simulink model "TST_AirHt_Ctl"  (R2016b)
settings: Solver=FixedStepDiscrete  StartTime=0.0  StopTime=simTime  FixedStep=sampleTime  RelTol=1e-3
values from neighbouring files (symbols this model uses):
  testCase = 1    [initTST_AirHt_Ctl_001.m]    (also in initTST_AirHt_Ctl_002.m = 2; initTST_AirHt_Ctl_003.m = 3; initTST_AirHt_Ctl_004.m = 4; initTST_AirHt_Ctl_005.m = 5)
libraries: simulink x53, UnitTest_Lib x26
(part 2 of 4)

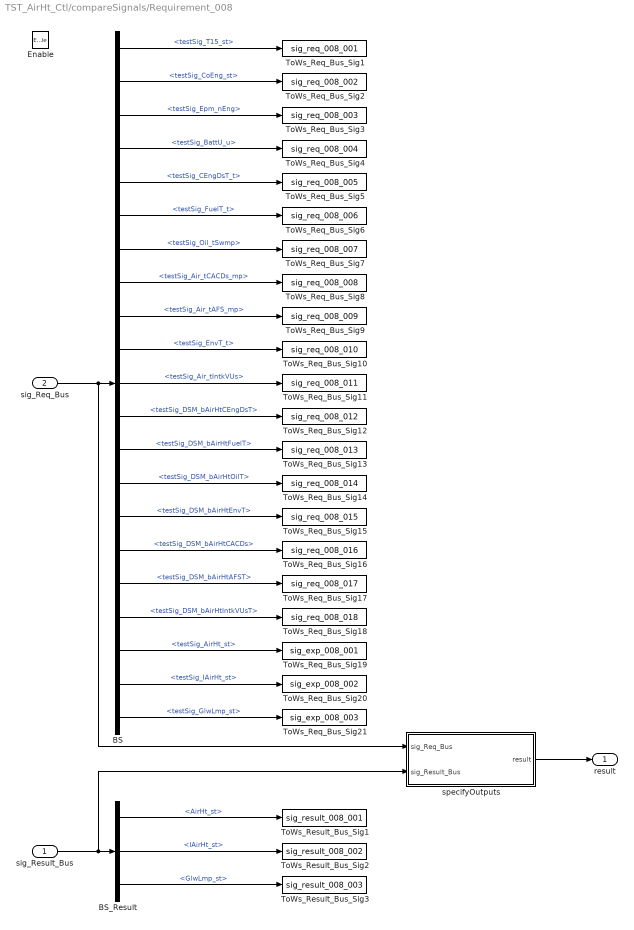
== system TST_AirHt_Ctl/compareSignals/Requirement_008 ==
  sig_Result_Bus : Inport
  sig_Req_Bus : Inport  Port=2
  Enable : EnablePort
  BS : BusSelector  OutputSignals=testSig_T15_st,testSig_CoEng_st,testSig_Epm_nEng,testSig_BattU_u,testSig_CEngDsT_t,testSig_FuelT_t,testSig_Oil_tSwmp,testSig_Air_tCACDs_mp,testSig_Air_tAFS_mp,testSig_EnvT_t,testSig_Air_tIntkVUs,testSig_DSM_bAirHtCEngDsT,testSig_DSM_bAirHtFuelT,testSig_DSM_bAirHtOilT,testSig_DSM_bAirHtEnvT,testSig_DSM_bAirHtCACDs,testSig_DSM_bAirHtAFST,testSig_DSM_bAirHtIntkVUsT,testSig_AirHt_st,testSig_IAirHt_st,testSig_GlwLmp_st
  BS_Result : BusSelector  OutputSignals=AirHt_st,IAirHt_st,GlwLmp_st
  ToWs_Req_Bus_Sig1 : ToWorkspace  VariableName=sig_req_008_001  SaveFormat=Structure With Time
  ToWs_Req_Bus_Sig10 : ToWorkspace  VariableName=sig_req_008_010  SaveFormat=Structure With Time
  ToWs_Req_Bus_Sig11 : ToWorkspace  VariableName=sig_req_008_011  SaveFormat=Structure With Time
  ToWs_Req_Bus_Sig12 : ToWorkspace  VariableName=sig_req_008_012  SaveFormat=Structure With Time
  ToWs_Req_Bus_Sig13 : ToWorkspace  VariableName=sig_req_008_013  SaveFormat=Structure With Time
  ToWs_Req_Bus_Sig14 : ToWorkspace  VariableName=sig_req_008_014  SaveFormat=Structure With Time
  ToWs_Req_Bus_Sig15 : ToWorkspace  VariableName=sig_req_008_015  SaveFormat=Structure With Time
  ToWs_Req_Bus_Sig16 : ToWorkspace  VariableName=sig_req_008_016  SaveFormat=Structure With Time
  ToWs_Req_Bus_Sig17 : ToWorkspace  VariableName=sig_req_008_017  SaveFormat=Structure With Time
  ToWs_Req_Bus_Sig18 : ToWorkspace  VariableName=sig_req_008_018  SaveFormat=Structure With Time
  ToWs_Req_Bus_Sig19 : ToWorkspace  VariableName=sig_exp_008_001  SaveFormat=Structure With Time
  ToWs_Req_Bus_Sig2 : ToWorkspace  VariableName=sig_req_008_002  SaveFormat=Structure With Time
  ToWs_Req_Bus_Sig20 : ToWorkspace  VariableName=sig_exp_008_002  SaveFormat=Structure With Time
  ToWs_Req_Bus_Sig21 : ToWorkspace  VariableName=sig_exp_008_003  SaveFormat=Structure With Time
  ToWs_Req_Bus_Sig3 : ToWorkspace  VariableName=sig_req_008_003  SaveFormat=Structure With Time
  ToWs_Req_Bus_Sig4 : ToWorkspace  VariableName=sig_req_008_004  SaveFormat=Structure With Time
  ToWs_Req_Bus_Sig5 : ToWorkspace  VariableName=sig_req_008_005  SaveFormat=Structure With Time
  ToWs_Req_Bus_Sig6 : ToWorkspace  VariableName=sig_req_008_006  SaveFormat=Structure With Time
  ToWs_Req_Bus_Sig7 : ToWorkspace  VariableName=sig_req_008_007  SaveFormat=Structure With Time
  ToWs_Req_Bus_Sig8 : ToWorkspace  VariableName=sig_req_008_008  SaveFormat=Structure With Time
  ToWs_Req_Bus_Sig9 : ToWorkspace  VariableName=sig_req_008_009  SaveFormat=Structure With Time
  ToWs_Result_Bus_Sig1 : ToWorkspace  VariableName=sig_result_008_001  SaveFormat=Structure With Time
  ToWs_Result_Bus_Sig2 : ToWorkspace  VariableName=sig_result_008_002  SaveFormat=Structure With Time
  ToWs_Result_Bus_Sig3 : ToWorkspace  VariableName=sig_result_008_003  SaveFormat=Structure With Time
  specifyOutputs : Subsystem
  result : Outport
  wires:
  sig_Req_Bus/1 -> BS/1, specifyOutputs/1(sig_Req_Bus)
  BS/1 -> ToWs_Req_Bus_Sig1/1  "<testSig_T15_st>"
  BS/2 -> ToWs_Req_Bus_Sig2/1  "<testSig_CoEng_st>"
  BS/3 -> ToWs_Req_Bus_Sig3/1  "<testSig_Epm_nEng>"
  BS/4 -> ToWs_Req_Bus_Sig4/1  "<testSig_BattU_u>"
  BS/5 -> ToWs_Req_Bus_Sig5/1  "<testSig_CEngDsT_t>"
  BS/6 -> ToWs_Req_Bus_Sig6/1  "<testSig_FuelT_t>"
  BS/7 -> ToWs_Req_Bus_Sig7/1  "<testSig_Oil_tSwmp>"
  BS/8 -> ToWs_Req_Bus_Sig8/1  "<testSig_Air_tCACDs_mp>"
  BS/9 -> ToWs_Req_Bus_Sig9/1  "<testSig_Air_tAFS_mp>"
  BS/10 -> ToWs_Req_Bus_Sig10/1  "<testSig_EnvT_t>"
  BS/11 -> ToWs_Req_Bus_Sig11/1  "<testSig_Air_tIntkVUs>"
  BS/12 -> ToWs_Req_Bus_Sig12/1  "<testSig_DSM_bAirHtCEngDsT>"
  BS/13 -> ToWs_Req_Bus_Sig13/1  "<testSig_DSM_bAirHtFuelT>"
  BS/14 -> ToWs_Req_Bus_Sig14/1  "<testSig_DSM_bAirHtOilT>"
  BS/15 -> ToWs_Req_Bus_Sig15/1  "<testSig_DSM_bAirHtEnvT>"
  BS/16 -> ToWs_Req_Bus_Sig16/1  "<testSig_DSM_bAirHtCACDs>"
  BS/17 -> ToWs_Req_Bus_Sig17/1  "<testSig_DSM_bAirHtAFST>"
  BS/18 -> ToWs_Req_Bus_Sig18/1  "<testSig_DSM_bAirHtIntkVUsT>"
  BS/19 -> ToWs_Req_Bus_Sig19/1  "<testSig_AirHt_st>"
  BS/20 -> ToWs_Req_Bus_Sig20/1  "<testSig_IAirHt_st>"
  BS/21 -> ToWs_Req_Bus_Sig21/1  "<testSig_GlwLmp_st>"
  sig_Result_Bus/1 -> BS_Result/1, specifyOutputs/2(sig_Result_Bus)
  BS_Result/1 -> ToWs_Result_Bus_Sig1/1  "<AirHt_st>"
  BS_Result/2 -> ToWs_Result_Bus_Sig2/1  "<IAirHt_st>"
  BS_Result/3 -> ToWs_Result_Bus_Sig3/1  "<GlwLmp_st>"
  specifyOutputs/1(result) -> result/1

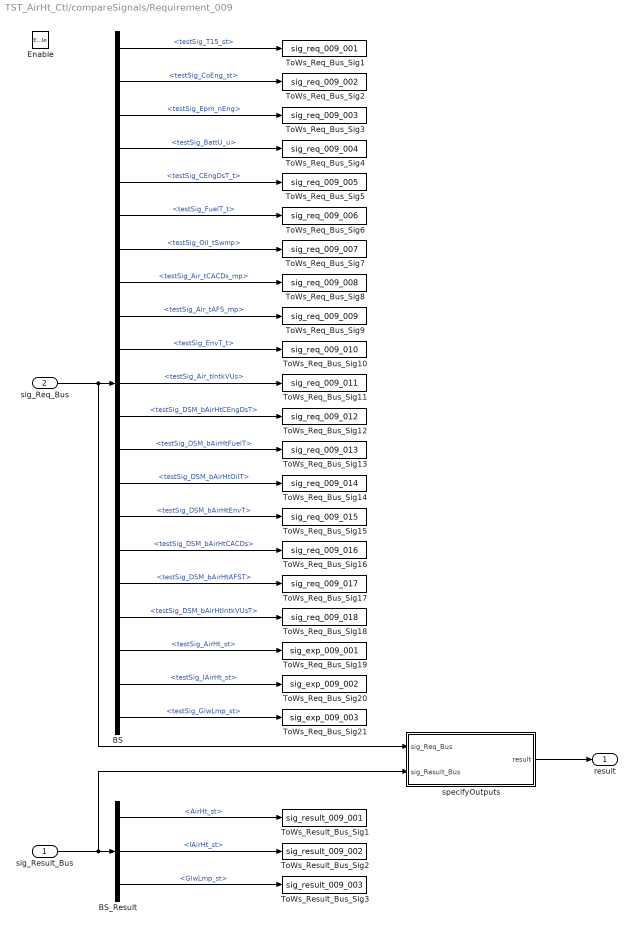
== system TST_AirHt_Ctl/compareSignals/Requirement_009 ==
  sig_Result_Bus : Inport
  sig_Req_Bus : Inport  Port=2
  Enable : EnablePort
  BS : BusSelector  OutputSignals=testSig_T15_st,testSig_CoEng_st,testSig_Epm_nEng,testSig_BattU_u,testSig_CEngDsT_t,testSig_FuelT_t,testSig_Oil_tSwmp,testSig_Air_tCACDs_mp,testSig_Air_tAFS_mp,testSig_EnvT_t,testSig_Air_tIntkVUs,testSig_DSM_bAirHtCEngDsT,testSig_DSM_bAirHtFuelT,testSig_DSM_bAirHtOilT,testSig_DSM_bAirHtEnvT,testSig_DSM_bAirHtCACDs,testSig_DSM_bAirHtAFST,testSig_DSM_bAirHtIntkVUsT,testSig_AirHt_st,testSig_IAirHt_st,testSig_GlwLmp_st
  BS_Result : BusSelector  OutputSignals=AirHt_st,IAirHt_st,GlwLmp_st
  ToWs_Req_Bus_Sig1 : ToWorkspace  VariableName=sig_req_009_001  SaveFormat=Structure With Time
  ToWs_Req_Bus_Sig10 : ToWorkspace  VariableName=sig_req_009_010  SaveFormat=Structure With Time
  ToWs_Req_Bus_Sig11 : ToWorkspace  VariableName=sig_req_009_011  SaveFormat=Structure With Time
  ToWs_Req_Bus_Sig12 : ToWorkspace  VariableName=sig_req_009_012  SaveFormat=Structure With Time
  ToWs_Req_Bus_Sig13 : ToWorkspace  VariableName=sig_req_009_013  SaveFormat=Structure With Time
  ToWs_Req_Bus_Sig14 : ToWorkspace  VariableName=sig_req_009_014  SaveFormat=Structure With Time
  ToWs_Req_Bus_Sig15 : ToWorkspace  VariableName=sig_req_009_015  SaveFormat=Structure With Time
  ToWs_Req_Bus_Sig16 : ToWorkspace  VariableName=sig_req_009_016  SaveFormat=Structure With Time
  ToWs_Req_Bus_Sig17 : ToWorkspace  VariableName=sig_req_009_017  SaveFormat=Structure With Time
  ToWs_Req_Bus_Sig18 : ToWorkspace  VariableName=sig_req_009_018  SaveFormat=Structure With Time
  ToWs_Req_Bus_Sig19 : ToWorkspace  VariableName=sig_exp_009_001  SaveFormat=Structure With Time
  ToWs_Req_Bus_Sig2 : ToWorkspace  VariableName=sig_req_009_002  SaveFormat=Structure With Time
  ToWs_Req_Bus_Sig20 : ToWorkspace  VariableName=sig_exp_009_002  SaveFormat=Structure With Time
  ToWs_Req_Bus_Sig21 : ToWorkspace  VariableName=sig_exp_009_003  SaveFormat=Structure With Time
  ToWs_Req_Bus_Sig3 : ToWorkspace  VariableName=sig_req_009_003  SaveFormat=Structure With Time
  ToWs_Req_Bus_Sig4 : ToWorkspace  VariableName=sig_req_009_004  SaveFormat=Structure With Time
  ToWs_Req_Bus_Sig5 : ToWorkspace  VariableName=sig_req_009_005  SaveFormat=Structure With Time
  ToWs_Req_Bus_Sig6 : ToWorkspace  VariableName=sig_req_009_006  SaveFormat=Structure With Time
  ToWs_Req_Bus_Sig7 : ToWorkspace  VariableName=sig_req_009_007  SaveFormat=Structure With Time
  ToWs_Req_Bus_Sig8 : ToWorkspace  VariableName=sig_req_009_008  SaveFormat=Structure With Time
  ToWs_Req_Bus_Sig9 : ToWorkspace  VariableName=sig_req_009_009  SaveFormat=Structure With Time
  ToWs_Result_Bus_Sig1 : ToWorkspace  VariableName=sig_result_009_001  SaveFormat=Structure With Time
  ToWs_Result_Bus_Sig2 : ToWorkspace  VariableName=sig_result_009_002  SaveFormat=Structure With Time
  ToWs_Result_Bus_Sig3 : ToWorkspace  VariableName=sig_result_009_003  SaveFormat=Structure With Time
  specifyOutputs : Subsystem
  result : Outport
  wires:
  sig_Req_Bus/1 -> BS/1, specifyOutputs/1(sig_Req_Bus)
  BS/1 -> ToWs_Req_Bus_Sig1/1  "<testSig_T15_st>"
  BS/2 -> ToWs_Req_Bus_Sig2/1  "<testSig_CoEng_st>"
  BS/3 -> ToWs_Req_Bus_Sig3/1  "<testSig_Epm_nEng>"
  BS/4 -> ToWs_Req_Bus_Sig4/1  "<testSig_BattU_u>"
  BS/5 -> ToWs_Req_Bus_Sig5/1  "<testSig_CEngDsT_t>"
  BS/6 -> ToWs_Req_Bus_Sig6/1  "<testSig_FuelT_t>"
  BS/7 -> ToWs_Req_Bus_Sig7/1  "<testSig_Oil_tSwmp>"
  BS/8 -> ToWs_Req_Bus_Sig8/1  "<testSig_Air_tCACDs_mp>"
  BS/9 -> ToWs_Req_Bus_Sig9/1  "<testSig_Air_tAFS_mp>"
  BS/10 -> ToWs_Req_Bus_Sig10/1  "<testSig_EnvT_t>"
  BS/11 -> ToWs_Req_Bus_Sig11/1  "<testSig_Air_tIntkVUs>"
  BS/12 -> ToWs_Req_Bus_Sig12/1  "<testSig_DSM_bAirHtCEngDsT>"
  BS/13 -> ToWs_Req_Bus_Sig13/1  "<testSig_DSM_bAirHtFuelT>"
  BS/14 -> ToWs_Req_Bus_Sig14/1  "<testSig_DSM_bAirHtOilT>"
  BS/15 -> ToWs_Req_Bus_Sig15/1  "<testSig_DSM_bAirHtEnvT>"
  BS/16 -> ToWs_Req_Bus_Sig16/1  "<testSig_DSM_bAirHtCACDs>"
  BS/17 -> ToWs_Req_Bus_Sig17/1  "<testSig_DSM_bAirHtAFST>"
  BS/18 -> ToWs_Req_Bus_Sig18/1  "<testSig_DSM_bAirHtIntkVUsT>"
  BS/19 -> ToWs_Req_Bus_Sig19/1  "<testSig_AirHt_st>"
  BS/20 -> ToWs_Req_Bus_Sig20/1  "<testSig_IAirHt_st>"
  BS/21 -> ToWs_Req_Bus_Sig21/1  "<testSig_GlwLmp_st>"
  sig_Result_Bus/1 -> BS_Result/1, specifyOutputs/2(sig_Result_Bus)
  BS_Result/1 -> ToWs_Result_Bus_Sig1/1  "<AirHt_st>"
  BS_Result/2 -> ToWs_Result_Bus_Sig2/1  "<IAirHt_st>"
  BS_Result/3 -> ToWs_Result_Bus_Sig3/1  "<GlwLmp_st>"
  specifyOutputs/1(result) -> result/1

== system TST_AirHt_Ctl/compareSignals/Requirement_010 ==
  sig_Result_Bus : Inport
  sig_Req_Bus : Inport  Port=2
  Enable : EnablePort
  BS : BusSelector  OutputSignals=testSig_T15_st,testSig_CoEng_st,testSig_Epm_nEng,testSig_BattU_u,testSig_CEngDsT_t,testSig_FuelT_t,testSig_Oil_tSwmp,testSig_Air_tCACDs_mp,testSig_Air_tAFS_mp,testSig_EnvT_t,testSig_Air_tIntkVUs,testSig_DSM_bAirHtCEngDsT,testSig_DSM_bAirHtFuelT,testSig_DSM_bAirHtOilT,testSig_DSM_bAirHtEnvT,testSig_DSM_bAirHtCACDs,testSig_DSM_bAirHtAFST,testSig_DSM_bAirHtIntkVUsT,testSig_AirHt_st,testSig_IAirHt_st,testSig_GlwLmp_st
  BS_Result : BusSelector  OutputSignals=AirHt_st,IAirHt_st,GlwLmp_st
  ToWs_Req_Bus_Sig1 : ToWorkspace  VariableName=sig_req_010_001  SaveFormat=Structure With Time
  ToWs_Req_Bus_Sig10 : ToWorkspace  VariableName=sig_req_010_010  SaveFormat=Structure With Time
  ToWs_Req_Bus_Sig11 : ToWorkspace  VariableName=sig_req_010_011  SaveFormat=Structure With Time
  ToWs_Req_Bus_Sig12 : ToWorkspace  VariableName=sig_req_010_012  SaveFormat=Structure With Time
  ToWs_Req_Bus_Sig13 : ToWorkspace  VariableName=sig_req_010_013  SaveFormat=Structure With Time
  ToWs_Req_Bus_Sig14 : ToWorkspace  VariableName=sig_req_010_014  SaveFormat=Structure With Time
  ToWs_Req_Bus_Sig15 : ToWorkspace  VariableName=sig_req_010_015  SaveFormat=Structure With Time
  ToWs_Req_Bus_Sig16 : ToWorkspace  VariableName=sig_req_010_016  SaveFormat=Structure With Time
  ToWs_Req_Bus_Sig17 : ToWorkspace  VariableName=sig_req_010_017  SaveFormat=Structure With Time
  ToWs_Req_Bus_Sig18 : ToWorkspace  VariableName=sig_req_010_018  SaveFormat=Structure With Time
  ToWs_Req_Bus_Sig19 : ToWorkspace  VariableName=sig_exp_010_001  SaveFormat=Structure With Time
  ToWs_Req_Bus_Sig2 : ToWorkspace  VariableName=sig_req_010_002  SaveFormat=Structure With Time
  ToWs_Req_Bus_Sig20 : ToWorkspace  VariableName=sig_exp_010_002  SaveFormat=Structure With Time
  ToWs_Req_Bus_Sig21 : ToWorkspace  VariableName=sig_exp_010_003  SaveFormat=Structure With Time
  ToWs_Req_Bus_Sig3 : ToWorkspace  VariableName=sig_req_010_003  SaveFormat=Structure With Time
  ToWs_Req_Bus_Sig4 : ToWorkspace  VariableName=sig_req_010_004  SaveFormat=Structure With Time
  ToWs_Req_Bus_Sig5 : ToWorkspace  VariableName=sig_req_010_005  SaveFormat=Structure With Time
  ToWs_Req_Bus_Sig6 : ToWorkspace  VariableName=sig_req_010_006  SaveFormat=Structure With Time
  ToWs_Req_Bus_Sig7 : ToWorkspace  VariableName=sig_req_010_007  SaveFormat=Structure With Time
  ToWs_Req_Bus_Sig8 : ToWorkspace  VariableName=sig_req_010_008  SaveFormat=Structure With Time
  ToWs_Req_Bus_Sig9 : ToWorkspace  VariableName=sig_req_010_009  SaveFormat=Structure With Time
  ToWs_Result_Bus_Sig1 : ToWorkspace  VariableName=sig_result_010_001  SaveFormat=Structure With Time
  ToWs_Result_Bus_Sig2 : ToWorkspace  VariableName=sig_result_010_002  SaveFormat=Structure With Time
  ToWs_Result_Bus_Sig3 : ToWorkspace  VariableName=sig_result_010_003  SaveFormat=Structure With Time
  specifyOutputs : Subsystem
  result : Outport
  wires:
  sig_Req_Bus/1 -> BS/1, specifyOutputs/1(sig_Req_Bus)
  BS/1 -> ToWs_Req_Bus_Sig1/1  "<testSig_T15_st>"
  BS/2 -> ToWs_Req_Bus_Sig2/1  "<testSig_CoEng_st>"
  BS/3 -> ToWs_Req_Bus_Sig3/1  "<testSig_Epm_nEng>"
  BS/4 -> ToWs_Req_Bus_Sig4/1  "<testSig_BattU_u>"
  BS/5 -> ToWs_Req_Bus_Sig5/1  "<testSig_CEngDsT_t>"
  BS/6 -> ToWs_Req_Bus_Sig6/1  "<testSig_FuelT_t>"
  BS/7 -> ToWs_Req_Bus_Sig7/1  "<testSig_Oil_tSwmp>"
  BS/8 -> ToWs_Req_Bus_Sig8/1  "<testSig_Air_tCACDs_mp>"
  BS/9 -> ToWs_Req_Bus_Sig9/1  "<testSig_Air_tAFS_mp>"
  BS/10 -> ToWs_Req_Bus_Sig10/1  "<testSig_EnvT_t>"
  BS/11 -> ToWs_Req_Bus_Sig11/1  "<testSig_Air_tIntkVUs>"
  BS/12 -> ToWs_Req_Bus_Sig12/1  "<testSig_DSM_bAirHtCEngDsT>"
  BS/13 -> ToWs_Req_Bus_Sig13/1  "<testSig_DSM_bAirHtFuelT>"
  BS/14 -> ToWs_Req_Bus_Sig14/1  "<testSig_DSM_bAirHtOilT>"
  BS/15 -> ToWs_Req_Bus_Sig15/1  "<testSig_DSM_bAirHtEnvT>"
  BS/16 -> ToWs_Req_Bus_Sig16/1  "<testSig_DSM_bAirHtCACDs>"
  BS/17 -> ToWs_Req_Bus_Sig17/1  "<testSig_DSM_bAirHtAFST>"
  BS/18 -> ToWs_Req_Bus_Sig18/1  "<testSig_DSM_bAirHtIntkVUsT>"
  BS/19 -> ToWs_Req_Bus_Sig19/1  "<testSig_AirHt_st>"
  BS/20 -> ToWs_Req_Bus_Sig20/1  "<testSig_IAirHt_st>"
  BS/21 -> ToWs_Req_Bus_Sig21/1  "<testSig_GlwLmp_st>"
  sig_Result_Bus/1 -> BS_Result/1, specifyOutputs/2(sig_Result_Bus)
  BS_Result/1 -> ToWs_Result_Bus_Sig1/1  "<AirHt_st>"
  BS_Result/2 -> ToWs_Result_Bus_Sig2/1  "<IAirHt_st>"
  BS_Result/3 -> ToWs_Result_Bus_Sig3/1  "<GlwLmp_st>"
  specifyOutputs/1(result) -> result/1

== system TST_AirHt_Ctl/compareSignals/Requirement_011 ==
  sig_Result_Bus : Inport
  sig_Req_Bus : Inport  Port=2
  Enable : EnablePort
  BS : BusSelector  OutputSignals=testSig_T15_st,testSig_CoEng_st,testSig_Epm_nEng,testSig_BattU_u,testSig_CEngDsT_t,testSig_FuelT_t,testSig_Oil_tSwmp,testSig_Air_tCACDs_mp,testSig_Air_tAFS_mp,testSig_EnvT_t,testSig_Air_tIntkVUs,testSig_DSM_bAirHtCEngDsT,testSig_DSM_bAirHtFuelT,testSig_DSM_bAirHtOilT,testSig_DSM_bAirHtEnvT,testSig_DSM_bAirHtCACDs,testSig_DSM_bAirHtAFST,testSig_DSM_bAirHtIntkVUsT,testSig_AirHt_st,testSig_IAirHt_st,testSig_GlwLmp_st
  BS_Result : BusSelector  OutputSignals=AirHt_st,IAirHt_st,GlwLmp_st
  ToWs_Req_Bus_Sig1 : ToWorkspace  VariableName=sig_req_011_001  SaveFormat=Structure With Time
  ToWs_Req_Bus_Sig10 : ToWorkspace  VariableName=sig_req_011_010  SaveFormat=Structure With Time
  ToWs_Req_Bus_Sig11 : ToWorkspace  VariableName=sig_req_011_011  SaveFormat=Structure With Time
  ToWs_Req_Bus_Sig12 : ToWorkspace  VariableName=sig_req_011_012  SaveFormat=Structure With Time
  ToWs_Req_Bus_Sig13 : ToWorkspace  VariableName=sig_req_011_013  SaveFormat=Structure With Time
  ToWs_Req_Bus_Sig14 : ToWorkspace  VariableName=sig_req_011_014  SaveFormat=Structure With Time
  ToWs_Req_Bus_Sig15 : ToWorkspace  VariableName=sig_req_011_015  SaveFormat=Structure With Time
  ToWs_Req_Bus_Sig16 : ToWorkspace  VariableName=sig_req_011_016  SaveFormat=Structure With Time
  ToWs_Req_Bus_Sig17 : ToWorkspace  VariableName=sig_req_011_017  SaveFormat=Structure With Time
  ToWs_Req_Bus_Sig18 : ToWorkspace  VariableName=sig_req_011_018  SaveFormat=Structure With Time
  ToWs_Req_Bus_Sig19 : ToWorkspace  VariableName=sig_exp_011_001  SaveFormat=Structure With Time
  ToWs_Req_Bus_Sig2 : ToWorkspace  VariableName=sig_req_011_002  SaveFormat=Structure With Time
  ToWs_Req_Bus_Sig20 : ToWorkspace  VariableName=sig_exp_011_002  SaveFormat=Structure With Time
  ToWs_Req_Bus_Sig21 : ToWorkspace  VariableName=sig_exp_011_003  SaveFormat=Structure With Time
  ToWs_Req_Bus_Sig3 : ToWorkspace  VariableName=sig_req_011_003  SaveFormat=Structure With Time
  ToWs_Req_Bus_Sig4 : ToWorkspace  VariableName=sig_req_011_004  SaveFormat=Structure With Time
  ToWs_Req_Bus_Sig5 : ToWorkspace  VariableName=sig_req_011_005  SaveFormat=Structure With Time
  ToWs_Req_Bus_Sig6 : ToWorkspace  VariableName=sig_req_011_006  SaveFormat=Structure With Time
  ToWs_Req_Bus_Sig7 : ToWorkspace  VariableName=sig_req_011_007  SaveFormat=Structure With Time
  ToWs_Req_Bus_Sig8 : ToWorkspace  VariableName=sig_req_011_008  SaveFormat=Structure With Time
  ToWs_Req_Bus_Sig9 : ToWorkspace  VariableName=sig_req_011_009  SaveFormat=Structure With Time
  ToWs_Result_Bus_Sig1 : ToWorkspace  VariableName=sig_result_011_001  SaveFormat=Structure With Time
  ToWs_Result_Bus_Sig2 : ToWorkspace  VariableName=sig_result_011_002  SaveFormat=Structure With Time
  ToWs_Result_Bus_Sig3 : ToWorkspace  VariableName=sig_result_011_003  SaveFormat=Structure With Time
  specifyOutputs : Subsystem
  result : Outport
  wires:
  sig_Req_Bus/1 -> BS/1, specifyOutputs/1(sig_Req_Bus)
  BS/1 -> ToWs_Req_Bus_Sig1/1  "<testSig_T15_st>"
  BS/2 -> ToWs_Req_Bus_Sig2/1  "<testSig_CoEng_st>"
  BS/3 -> ToWs_Req_Bus_Sig3/1  "<testSig_Epm_nEng>"
  BS/4 -> ToWs_Req_Bus_Sig4/1  "<testSig_BattU_u>"
  BS/5 -> ToWs_Req_Bus_Sig5/1  "<testSig_CEngDsT_t>"
  BS/6 -> ToWs_Req_Bus_Sig6/1  "<testSig_FuelT_t>"
  BS/7 -> ToWs_Req_Bus_Sig7/1  "<testSig_Oil_tSwmp>"
  BS/8 -> ToWs_Req_Bus_Sig8/1  "<testSig_Air_tCACDs_mp>"
  BS/9 -> ToWs_Req_Bus_Sig9/1  "<testSig_Air_tAFS_mp>"
  BS/10 -> ToWs_Req_Bus_Sig10/1  "<testSig_EnvT_t>"
  BS/11 -> ToWs_Req_Bus_Sig11/1  "<testSig_Air_tIntkVUs>"
  BS/12 -> ToWs_Req_Bus_Sig12/1  "<testSig_DSM_bAirHtCEngDsT>"
  BS/13 -> ToWs_Req_Bus_Sig13/1  "<testSig_DSM_bAirHtFuelT>"
  BS/14 -> ToWs_Req_Bus_Sig14/1  "<testSig_DSM_bAirHtOilT>"
  BS/15 -> ToWs_Req_Bus_Sig15/1  "<testSig_DSM_bAirHtEnvT>"
  BS/16 -> ToWs_Req_Bus_Sig16/1  "<testSig_DSM_bAirHtCACDs>"
  BS/17 -> ToWs_Req_Bus_Sig17/1  "<testSig_DSM_bAirHtAFST>"
  BS/18 -> ToWs_Req_Bus_Sig18/1  "<testSig_DSM_bAirHtIntkVUsT>"
  BS/19 -> ToWs_Req_Bus_Sig19/1  "<testSig_AirHt_st>"
  BS/20 -> ToWs_Req_Bus_Sig20/1  "<testSig_IAirHt_st>"
  BS/21 -> ToWs_Req_Bus_Sig21/1  "<testSig_GlwLmp_st>"
  sig_Result_Bus/1 -> BS_Result/1, specifyOutputs/2(sig_Result_Bus)
  BS_Result/1 -> ToWs_Result_Bus_Sig1/1  "<AirHt_st>"
  BS_Result/2 -> ToWs_Result_Bus_Sig2/1  "<IAirHt_st>"
  BS_Result/3 -> ToWs_Result_Bus_Sig3/1  "<GlwLmp_st>"
  specifyOutputs/1(result) -> result/1

== system TST_AirHt_Ctl/compareSignals/Requirement_012 ==
  sig_Result_Bus : Inport
  sig_Req_Bus : Inport  Port=2
  Enable : EnablePort
  BS : BusSelector  OutputSignals=testSig_T15_st,testSig_CoEng_st,testSig_Epm_nEng,testSig_BattU_u,testSig_CEngDsT_t,testSig_FuelT_t,testSig_Oil_tSwmp,testSig_Air_tCACDs_mp,testSig_Air_tAFS_mp,testSig_EnvT_t,testSig_Air_tIntkVUs,testSig_DSM_bAirHtCEngDsT,testSig_DSM_bAirHtFuelT,testSig_DSM_bAirHtOilT,testSig_DSM_bAirHtEnvT,testSig_DSM_bAirHtCACDs,testSig_DSM_bAirHtAFST,testSig_DSM_bAirHtIntkVUsT,testSig_AirHt_st,testSig_IAirHt_st,testSig_GlwLmp_st
  BS_Result : BusSelector  OutputSignals=AirHt_st,IAirHt_st,GlwLmp_st
  ToWs_Req_Bus_Sig1 : ToWorkspace  VariableName=sig_req_012_001  SaveFormat=Structure With Time
  ToWs_Req_Bus_Sig10 : ToWorkspace  VariableName=sig_req_012_010  SaveFormat=Structure With Time
  ToWs_Req_Bus_Sig11 : ToWorkspace  VariableName=sig_req_012_011  SaveFormat=Structure With Time
  ToWs_Req_Bus_Sig12 : ToWorkspace  VariableName=sig_req_012_012  SaveFormat=Structure With Time
  ToWs_Req_Bus_Sig13 : ToWorkspace  VariableName=sig_req_012_013  SaveFormat=Structure With Time
  ToWs_Req_Bus_Sig14 : ToWorkspace  VariableName=sig_req_012_014  SaveFormat=Structure With Time
  ToWs_Req_Bus_Sig15 : ToWorkspace  VariableName=sig_req_012_015  SaveFormat=Structure With Time
  ToWs_Req_Bus_Sig16 : ToWorkspace  VariableName=sig_req_012_016  SaveFormat=Structure With Time
  ToWs_Req_Bus_Sig17 : ToWorkspace  VariableName=sig_req_012_017  SaveFormat=Structure With Time
  ToWs_Req_Bus_Sig18 : ToWorkspace  VariableName=sig_req_012_018  SaveFormat=Structure With Time
  ToWs_Req_Bus_Sig19 : ToWorkspace  VariableName=sig_exp_012_001  SaveFormat=Structure With Time
  ToWs_Req_Bus_Sig2 : ToWorkspace  VariableName=sig_req_012_002  SaveFormat=Structure With Time
  ToWs_Req_Bus_Sig20 : ToWorkspace  VariableName=sig_exp_012_002  SaveFormat=Structure With Time
  ToWs_Req_Bus_Sig21 : ToWorkspace  VariableName=sig_exp_012_003  SaveFormat=Structure With Time
  ToWs_Req_Bus_Sig3 : ToWorkspace  VariableName=sig_req_012_003  SaveFormat=Structure With Time
  ToWs_Req_Bus_Sig4 : ToWorkspace  VariableName=sig_req_012_004  SaveFormat=Structure With Time
  ToWs_Req_Bus_Sig5 : ToWorkspace  VariableName=sig_req_012_005  SaveFormat=Structure With Time
  ToWs_Req_Bus_Sig6 : ToWorkspace  VariableName=sig_req_012_006  SaveFormat=Structure With Time
  ToWs_Req_Bus_Sig7 : ToWorkspace  VariableName=sig_req_012_007  SaveFormat=Structure With Time
  ToWs_Req_Bus_Sig8 : ToWorkspace  VariableName=sig_req_012_008  SaveFormat=Structure With Time
  ToWs_Req_Bus_Sig9 : ToWorkspace  VariableName=sig_req_012_009  SaveFormat=Structure With Time
  ToWs_Result_Bus_Sig1 : ToWorkspace  VariableName=sig_result_012_001  SaveFormat=Structure With Time
  ToWs_Result_Bus_Sig2 : ToWorkspace  VariableName=sig_result_012_002  SaveFormat=Structure With Time
  ToWs_Result_Bus_Sig3 : ToWorkspace  VariableName=sig_result_012_003  SaveFormat=Structure With Time
  specifyOutputs : Subsystem
  result : Outport
  wires:
  sig_Req_Bus/1 -> BS/1, specifyOutputs/1(sig_Req_Bus)
  BS/1 -> ToWs_Req_Bus_Sig1/1  "<testSig_T15_st>"
  BS/2 -> ToWs_Req_Bus_Sig2/1  "<testSig_CoEng_st>"
  BS/3 -> ToWs_Req_Bus_Sig3/1  "<testSig_Epm_nEng>"
  BS/4 -> ToWs_Req_Bus_Sig4/1  "<testSig_BattU_u>"
  BS/5 -> ToWs_Req_Bus_Sig5/1  "<testSig_CEngDsT_t>"
  BS/6 -> ToWs_Req_Bus_Sig6/1  "<testSig_FuelT_t>"
  BS/7 -> ToWs_Req_Bus_Sig7/1  "<testSig_Oil_tSwmp>"
  BS/8 -> ToWs_Req_Bus_Sig8/1  "<testSig_Air_tCACDs_mp>"
  BS/9 -> ToWs_Req_Bus_Sig9/1  "<testSig_Air_tAFS_mp>"
  BS/10 -> ToWs_Req_Bus_Sig10/1  "<testSig_EnvT_t>"
  BS/11 -> ToWs_Req_Bus_Sig11/1  "<testSig_Air_tIntkVUs>"
  BS/12 -> ToWs_Req_Bus_Sig12/1  "<testSig_DSM_bAirHtCEngDsT>"
  BS/13 -> ToWs_Req_Bus_Sig13/1  "<testSig_DSM_bAirHtFuelT>"
  BS/14 -> ToWs_Req_Bus_Sig14/1  "<testSig_DSM_bAirHtOilT>"
  BS/15 -> ToWs_Req_Bus_Sig15/1  "<testSig_DSM_bAirHtEnvT>"
  BS/16 -> ToWs_Req_Bus_Sig16/1  "<testSig_DSM_bAirHtCACDs>"
  BS/17 -> ToWs_Req_Bus_Sig17/1  "<testSig_DSM_bAirHtAFST>"
  BS/18 -> ToWs_Req_Bus_Sig18/1  "<testSig_DSM_bAirHtIntkVUsT>"
  BS/19 -> ToWs_Req_Bus_Sig19/1  "<testSig_AirHt_st>"
  BS/20 -> ToWs_Req_Bus_Sig20/1  "<testSig_IAirHt_st>"
  BS/21 -> ToWs_Req_Bus_Sig21/1  "<testSig_GlwLmp_st>"
  sig_Result_Bus/1 -> BS_Result/1, specifyOutputs/2(sig_Result_Bus)
  BS_Result/1 -> ToWs_Result_Bus_Sig1/1  "<AirHt_st>"
  BS_Result/2 -> ToWs_Result_Bus_Sig2/1  "<IAirHt_st>"
  BS_Result/3 -> ToWs_Result_Bus_Sig3/1  "<GlwLmp_st>"
  specifyOutputs/1(result) -> result/1

== system TST_AirHt_Ctl/compareSignals/Requirement_013 ==
  sig_Result_Bus : Inport
  sig_Req_Bus : Inport  Port=2
  Enable : EnablePort
  BS : BusSelector  OutputSignals=testSig_T15_st,testSig_CoEng_st,testSig_Epm_nEng,testSig_BattU_u,testSig_CEngDsT_t,testSig_FuelT_t,testSig_Oil_tSwmp,testSig_Air_tCACDs_mp,testSig_Air_tAFS_mp,testSig_EnvT_t,testSig_Air_tIntkVUs,testSig_DSM_bAirHtCEngDsT,testSig_DSM_bAirHtFuelT,testSig_DSM_bAirHtOilT,testSig_DSM_bAirHtEnvT,testSig_DSM_bAirHtCACDs,testSig_DSM_bAirHtAFST,testSig_DSM_bAirHtIntkVUsT,testSig_AirHt_st,testSig_IAirHt_st,testSig_GlwLmp_st
  BS_Result : BusSelector  OutputSignals=AirHt_st,IAirHt_st,GlwLmp_st
  ToWs_Req_Bus_Sig1 : ToWorkspace  VariableName=sig_req_013_001  SaveFormat=Structure With Time
  ToWs_Req_Bus_Sig10 : ToWorkspace  VariableName=sig_req_013_010  SaveFormat=Structure With Time
  ToWs_Req_Bus_Sig11 : ToWorkspace  VariableName=sig_req_013_011  SaveFormat=Structure With Time
  ToWs_Req_Bus_Sig12 : ToWorkspace  VariableName=sig_req_013_012  SaveFormat=Structure With Time
  ToWs_Req_Bus_Sig13 : ToWorkspace  VariableName=sig_req_013_013  SaveFormat=Structure With Time
  ToWs_Req_Bus_Sig14 : ToWorkspace  VariableName=sig_req_013_014  SaveFormat=Structure With Time
  ToWs_Req_Bus_Sig15 : ToWorkspace  VariableName=sig_req_013_015  SaveFormat=Structure With Time
  ToWs_Req_Bus_Sig16 : ToWorkspace  VariableName=sig_req_013_016  SaveFormat=Structure With Time
  ToWs_Req_Bus_Sig17 : ToWorkspace  VariableName=sig_req_013_017  SaveFormat=Structure With Time
  ToWs_Req_Bus_Sig18 : ToWorkspace  VariableName=sig_req_013_018  SaveFormat=Structure With Time
  ToWs_Req_Bus_Sig19 : ToWorkspace  VariableName=sig_exp_013_001  SaveFormat=Structure With Time
  ToWs_Req_Bus_Sig2 : ToWorkspace  VariableName=sig_req_013_002  SaveFormat=Structure With Time
  ToWs_Req_Bus_Sig20 : ToWorkspace  VariableName=sig_exp_013_002  SaveFormat=Structure With Time
  ToWs_Req_Bus_Sig21 : ToWorkspace  VariableName=sig_exp_013_003  SaveFormat=Structure With Time
  ToWs_Req_Bus_Sig3 : ToWorkspace  VariableName=sig_req_013_003  SaveFormat=Structure With Time
  ToWs_Req_Bus_Sig4 : ToWorkspace  VariableName=sig_req_013_004  SaveFormat=Structure With Time
  ToWs_Req_Bus_Sig5 : ToWorkspace  VariableName=sig_req_013_005  SaveFormat=Structure With Time
  ToWs_Req_Bus_Sig6 : ToWorkspace  VariableName=sig_req_013_006  SaveFormat=Structure With Time
  ToWs_Req_Bus_Sig7 : ToWorkspace  VariableName=sig_req_013_007  SaveFormat=Structure With Time
  ToWs_Req_Bus_Sig8 : ToWorkspace  VariableName=sig_req_013_008  SaveFormat=Structure With Time
  ToWs_Req_Bus_Sig9 : ToWorkspace  VariableName=sig_req_013_009  SaveFormat=Structure With Time
  ToWs_Result_Bus_Sig1 : ToWorkspace  VariableName=sig_result_013_001  SaveFormat=Structure With Time
  ToWs_Result_Bus_Sig2 : ToWorkspace  VariableName=sig_result_013_002  SaveFormat=Structure With Time
  ToWs_Result_Bus_Sig3 : ToWorkspace  VariableName=sig_result_013_003  SaveFormat=Structure With Time
  specifyOutputs : Subsystem
  result : Outport
  wires:
  sig_Req_Bus/1 -> BS/1, specifyOutputs/1(sig_Req_Bus)
  BS/1 -> ToWs_Req_Bus_Sig1/1  "<testSig_T15_st>"
  BS/2 -> ToWs_Req_Bus_Sig2/1  "<testSig_CoEng_st>"
  BS/3 -> ToWs_Req_Bus_Sig3/1  "<testSig_Epm_nEng>"
  BS/4 -> ToWs_Req_Bus_Sig4/1  "<testSig_BattU_u>"
  BS/5 -> ToWs_Req_Bus_Sig5/1  "<testSig_CEngDsT_t>"
  BS/6 -> ToWs_Req_Bus_Sig6/1  "<testSig_FuelT_t>"
  BS/7 -> ToWs_Req_Bus_Sig7/1  "<testSig_Oil_tSwmp>"
  BS/8 -> ToWs_Req_Bus_Sig8/1  "<testSig_Air_tCACDs_mp>"
  BS/9 -> ToWs_Req_Bus_Sig9/1  "<testSig_Air_tAFS_mp>"
  BS/10 -> ToWs_Req_Bus_Sig10/1  "<testSig_EnvT_t>"
  BS/11 -> ToWs_Req_Bus_Sig11/1  "<testSig_Air_tIntkVUs>"
  BS/12 -> ToWs_Req_Bus_Sig12/1  "<testSig_DSM_bAirHtCEngDsT>"
  BS/13 -> ToWs_Req_Bus_Sig13/1  "<testSig_DSM_bAirHtFuelT>"
  BS/14 -> ToWs_Req_Bus_Sig14/1  "<testSig_DSM_bAirHtOilT>"
  BS/15 -> ToWs_Req_Bus_Sig15/1  "<testSig_DSM_bAirHtEnvT>"
  BS/16 -> ToWs_Req_Bus_Sig16/1  "<testSig_DSM_bAirHtCACDs>"
  BS/17 -> ToWs_Req_Bus_Sig17/1  "<testSig_DSM_bAirHtAFST>"
  BS/18 -> ToWs_Req_Bus_Sig18/1  "<testSig_DSM_bAirHtIntkVUsT>"
  BS/19 -> ToWs_Req_Bus_Sig19/1  "<testSig_AirHt_st>"
  BS/20 -> ToWs_Req_Bus_Sig20/1  "<testSig_IAirHt_st>"
  BS/21 -> ToWs_Req_Bus_Sig21/1  "<testSig_GlwLmp_st>"
  sig_Result_Bus/1 -> BS_Result/1, specifyOutputs/2(sig_Result_Bus)
  BS_Result/1 -> ToWs_Result_Bus_Sig1/1  "<AirHt_st>"
  BS_Result/2 -> ToWs_Result_Bus_Sig2/1  "<IAirHt_st>"
  BS_Result/3 -> ToWs_Result_Bus_Sig3/1  "<GlwLmp_st>"
  specifyOutputs/1(result) -> result/1

== system TST_AirHt_Ctl/simulationInput/testSignals_R001 ==
  BC : BusCreator  Inputs=21
  spec_AirHt_st : FromWorkspace  VariableName=testSig_AirHt_st  Interpolate=off  OutputAfterFinalValue=Holding final value
  spec_Air_tAFS_mp : FromWorkspace  VariableName=testSig_Air_tAFS_mp  Interpolate=off  OutputAfterFinalValue=Holding final value
  spec_Air_tCACDs_mp : FromWorkspace  VariableName=testSig_Air_tCACDs_mp  Interpolate=off  OutputAfterFinalValue=Holding final value
  spec_Air_tIntkVUs : FromWorkspace  VariableName=testSig_Air_tIntkVUs  Interpolate=off  OutputAfterFinalValue=Holding final value
  spec_BattU_u : FromWorkspace  VariableName=testSig_BattU_u  Interpolate=off  OutputAfterFinalValue=Holding final value
  spec_CEngDsT_t : FromWorkspace  VariableName=testSig_CEngDsT_t  Interpolate=off  OutputAfterFinalValue=Holding final value
  spec_CoEng_st : FromWorkspace  VariableName=testSig_CoEng_st  Interpolate=off  OutputAfterFinalValue=Holding final value
  spec_DSM_bAirHtAFST : FromWorkspace  VariableName=testSig_DSM_bAirHtAFST  Interpolate=off  OutputAfterFinalValue=Holding final value
  spec_DSM_bAirHtCACDs : FromWorkspace  VariableName=testSig_DSM_bAirHtCACDs  Interpolate=off  OutputAfterFinalValue=Holding final value
  spec_DSM_bAirHtCEngDsT : FromWorkspace  VariableName=testSig_DSM_bAirHtCEngDsT  Interpolate=off  OutputAfterFinalValue=Holding final value
  spec_DSM_bAirHtEnvT : FromWorkspace  VariableName=testSig_DSM_bAirHtEnvT  Interpolate=off  OutputAfterFinalValue=Holding final value
  spec_DSM_bAirHtFuelT : FromWorkspace  VariableName=testSig_DSM_bAirHtFuelT  Interpolate=off  OutputAfterFinalValue=Holding final value
  spec_DSM_bAirHtIntkVUsT : FromWorkspace  VariableName=testSig_DSM_bAirHtIntkVUsT  Interpolate=off  OutputAfterFinalValue=Holding final value
  spec_DSM_bAirHtOilT : FromWorkspace  VariableName=testSig_DSM_bAirHtOilT  Interpolate=off  OutputAfterFinalValue=Holding final value
  spec_EnvT_t : FromWorkspace  VariableName=testSig_EnvT_t  Interpolate=off  OutputAfterFinalValue=Holding final value
  spec_Epm_nEng : FromWorkspace  VariableName=testSig_Epm_nEng  Interpolate=off  OutputAfterFinalValue=Holding final value
  spec_FuelT_t : FromWorkspace  VariableName=testSig_FuelT_t  Interpolate=off  OutputAfterFinalValue=Holding final value
  spec_GlwLmp_st : FromWorkspace  VariableName=testSig_GlwLmp_st  Interpolate=off  OutputAfterFinalValue=Holding final value
  spec_IAirHt_st : FromWorkspace  VariableName=testSig_IAirHt_st  Interpolate=off  OutputAfterFinalValue=Holding final value
  spec_Oil_tSwmp : FromWorkspace  VariableName=testSig_Oil_tSwmp  Interpolate=off  OutputAfterFinalValue=Holding final value
  spec_T15_st : FromWorkspace  VariableName=testSig_T15_st  Interpolate=off  OutputAfterFinalValue=Holding final value
  testSignals : Outport
  wires:
  BC/1 -> testSignals/1
  spec_T15_st/1 -> BC/1  "testSig_T15_st"
  spec_CoEng_st/1 -> BC/2  "testSig_CoEng_st"
  spec_Epm_nEng/1 -> BC/3  "testSig_Epm_nEng"
  spec_BattU_u/1 -> BC/4  "testSig_BattU_u"
  spec_CEngDsT_t/1 -> BC/5  "testSig_CEngDsT_t"
  spec_FuelT_t/1 -> BC/6  "testSig_FuelT_t"
  spec_Oil_tSwmp/1 -> BC/7  "testSig_Oil_tSwmp"
  spec_Air_tCACDs_mp/1 -> BC/8  "testSig_Air_tCACDs_mp"
  spec_Air_tAFS_mp/1 -> BC/9  "testSig_Air_tAFS_mp"
  spec_EnvT_t/1 -> BC/10  "testSig_EnvT_t"
  spec_Air_tIntkVUs/1 -> BC/11  "testSig_Air_tIntkVUs"
  spec_DSM_bAirHtCEngDsT/1 -> BC/12  "testSig_DSM_bAirHtCEngDsT"
  spec_DSM_bAirHtFuelT/1 -> BC/13  "testSig_DSM_bAirHtFuelT"
  spec_DSM_bAirHtOilT/1 -> BC/14  "testSig_DSM_bAirHtOilT"
  spec_DSM_bAirHtEnvT/1 -> BC/15  "testSig_DSM_bAirHtEnvT"
  spec_DSM_bAirHtCACDs/1 -> BC/16  "testSig_DSM_bAirHtCACDs"
  spec_DSM_bAirHtAFST/1 -> BC/17  "testSig_DSM_bAirHtAFST"
  spec_DSM_bAirHtIntkVUsT/1 -> BC/18  "testSig_DSM_bAirHtIntkVUsT"
  spec_AirHt_st/1 -> BC/19  "testSig_AirHt_st"
  spec_IAirHt_st/1 -> BC/20  "testSig_IAirHt_st"
  spec_GlwLmp_st/1 -> BC/21  "testSig_GlwLmp_st"

== system TST_AirHt_Ctl/simulationInput/testSignals_R002 ==
  BC : BusCreator  Inputs=21
  spec_AirHt_st : FromWorkspace  VariableName=testSig_AirHt_st  Interpolate=off  OutputAfterFinalValue=Holding final value
  spec_Air_tAFS_mp : FromWorkspace  VariableName=testSig_Air_tAFS_mp  Interpolate=off  OutputAfterFinalValue=Holding final value
  spec_Air_tCACDs_mp : FromWorkspace  VariableName=testSig_Air_tCACDs_mp  Interpolate=off  OutputAfterFinalValue=Holding final value
  spec_Air_tIntkVUs : FromWorkspace  VariableName=testSig_Air_tIntkVUs  Interpolate=off  OutputAfterFinalValue=Holding final value
  spec_BattU_u : FromWorkspace  VariableName=testSig_BattU_u  Interpolate=off  OutputAfterFinalValue=Holding final value
  spec_CEngDsT_t : FromWorkspace  VariableName=testSig_CEngDsT_t  Interpolate=off  OutputAfterFinalValue=Holding final value
  spec_CoEng_st : FromWorkspace  VariableName=testSig_CoEng_st  Interpolate=off  OutputAfterFinalValue=Holding final value
  spec_DSM_bAirHtAFST : FromWorkspace  VariableName=testSig_DSM_bAirHtAFST  Interpolate=off  OutputAfterFinalValue=Holding final value
  spec_DSM_bAirHtCACDs : FromWorkspace  VariableName=testSig_DSM_bAirHtCACDs  Interpolate=off  OutputAfterFinalValue=Holding final value
  spec_DSM_bAirHtCEngDsT : FromWorkspace  VariableName=testSig_DSM_bAirHtCEngDsT  Interpolate=off  OutputAfterFinalValue=Holding final value
  spec_DSM_bAirHtEnvT : FromWorkspace  VariableName=testSig_DSM_bAirHtEnvT  Interpolate=off  OutputAfterFinalValue=Holding final value
  spec_DSM_bAirHtFuelT : FromWorkspace  VariableName=testSig_DSM_bAirHtFuelT  Interpolate=off  OutputAfterFinalValue=Holding final value
  spec_DSM_bAirHtIntkVUsT : FromWorkspace  VariableName=testSig_DSM_bAirHtIntkVUsT  Interpolate=off  OutputAfterFinalValue=Holding final value
  spec_DSM_bAirHtOilT : FromWorkspace  VariableName=testSig_DSM_bAirHtOilT  Interpolate=off  OutputAfterFinalValue=Holding final value
  spec_EnvT_t : FromWorkspace  VariableName=testSig_EnvT_t  Interpolate=off  OutputAfterFinalValue=Holding final value
  spec_Epm_nEng : FromWorkspace  VariableName=testSig_Epm_nEng  Interpolate=off  OutputAfterFinalValue=Holding final value
  spec_FuelT_t : FromWorkspace  VariableName=testSig_FuelT_t  Interpolate=off  OutputAfterFinalValue=Holding final value
  spec_GlwLmp_st : FromWorkspace  VariableName=testSig_GlwLmp_st  Interpolate=off  OutputAfterFinalValue=Holding final value
  spec_IAirHt_st : FromWorkspace  VariableName=testSig_IAirHt_st  Interpolate=off  OutputAfterFinalValue=Holding final value
  spec_Oil_tSwmp : FromWorkspace  VariableName=testSig_Oil_tSwmp  Interpolate=off  OutputAfterFinalValue=Holding final value
  spec_T15_st : FromWorkspace  VariableName=testSig_T15_st  Interpolate=off  OutputAfterFinalValue=Holding final value
  testSignals : Outport
  wires:
  BC/1 -> testSignals/1
  spec_T15_st/1 -> BC/1  "testSig_T15_st"
  spec_CoEng_st/1 -> BC/2  "testSig_CoEng_st"
  spec_Epm_nEng/1 -> BC/3  "testSig_Epm_nEng"
  spec_BattU_u/1 -> BC/4  "testSig_BattU_u"
  spec_CEngDsT_t/1 -> BC/5  "testSig_CEngDsT_t"
  spec_FuelT_t/1 -> BC/6  "testSig_FuelT_t"
  spec_Oil_tSwmp/1 -> BC/7  "testSig_Oil_tSwmp"
  spec_Air_tCACDs_mp/1 -> BC/8  "testSig_Air_tCACDs_mp"
  spec_Air_tAFS_mp/1 -> BC/9  "testSig_Air_tAFS_mp"
  spec_EnvT_t/1 -> BC/10  "testSig_EnvT_t"
  spec_Air_tIntkVUs/1 -> BC/11  "testSig_Air_tIntkVUs"
  spec_DSM_bAirHtCEngDsT/1 -> BC/12  "testSig_DSM_bAirHtCEngDsT"
  spec_DSM_bAirHtFuelT/1 -> BC/13  "testSig_DSM_bAirHtFuelT"
  spec_DSM_bAirHtOilT/1 -> BC/14  "testSig_DSM_bAirHtOilT"
  spec_DSM_bAirHtEnvT/1 -> BC/15  "testSig_DSM_bAirHtEnvT"
  spec_DSM_bAirHtCACDs/1 -> BC/16  "testSig_DSM_bAirHtCACDs"
  spec_DSM_bAirHtAFST/1 -> BC/17  "testSig_DSM_bAirHtAFST"
  spec_DSM_bAirHtIntkVUsT/1 -> BC/18  "testSig_DSM_bAirHtIntkVUsT"
  spec_AirHt_st/1 -> BC/19  "testSig_AirHt_st"
  spec_IAirHt_st/1 -> BC/20  "testSig_IAirHt_st"
  spec_GlwLmp_st/1 -> BC/21  "testSig_GlwLmp_st"

== system TST_AirHt_Ctl/simulationInput/testSignals_R003 ==
  BC : BusCreator  Inputs=21
  spec_AirHt_st : FromWorkspace  VariableName=testSig_AirHt_st  Interpolate=off  OutputAfterFinalValue=Holding final value
  spec_Air_tAFS_mp : FromWorkspace  VariableName=testSig_Air_tAFS_mp  Interpolate=off  OutputAfterFinalValue=Holding final value
  spec_Air_tCACDs_mp : FromWorkspace  VariableName=testSig_Air_tCACDs_mp  Interpolate=off  OutputAfterFinalValue=Holding final value
  spec_Air_tIntkVUs : FromWorkspace  VariableName=testSig_Air_tIntkVUs  Interpolate=off  OutputAfterFinalValue=Holding final value
  spec_BattU_u : FromWorkspace  VariableName=testSig_BattU_u  Interpolate=off  OutputAfterFinalValue=Holding final value
  spec_CEngDsT_t : FromWorkspace  VariableName=testSig_CEngDsT_t  Interpolate=off  OutputAfterFinalValue=Holding final value
  spec_CoEng_st : FromWorkspace  VariableName=testSig_CoEng_st  Interpolate=off  OutputAfterFinalValue=Holding final value
  spec_DSM_bAirHtAFST : FromWorkspace  VariableName=testSig_DSM_bAirHtAFST  Interpolate=off  OutputAfterFinalValue=Holding final value
  spec_DSM_bAirHtCACDs : FromWorkspace  VariableName=testSig_DSM_bAirHtCACDs  Interpolate=off  OutputAfterFinalValue=Holding final value
  spec_DSM_bAirHtCEngDsT : FromWorkspace  VariableName=testSig_DSM_bAirHtCEngDsT  Interpolate=off  OutputAfterFinalValue=Holding final value
  spec_DSM_bAirHtEnvT : FromWorkspace  VariableName=testSig_DSM_bAirHtEnvT  Interpolate=off  OutputAfterFinalValue=Holding final value
  spec_DSM_bAirHtFuelT : FromWorkspace  VariableName=testSig_DSM_bAirHtFuelT  Interpolate=off  OutputAfterFinalValue=Holding final value
  spec_DSM_bAirHtIntkVUsT : FromWorkspace  VariableName=testSig_DSM_bAirHtIntkVUsT  Interpolate=off  OutputAfterFinalValue=Holding final value
  spec_DSM_bAirHtOilT : FromWorkspace  VariableName=testSig_DSM_bAirHtOilT  Interpolate=off  OutputAfterFinalValue=Holding final value
  spec_EnvT_t : FromWorkspace  VariableName=testSig_EnvT_t  Interpolate=off  OutputAfterFinalValue=Holding final value
  spec_Epm_nEng : FromWorkspace  VariableName=testSig_Epm_nEng  Interpolate=off  OutputAfterFinalValue=Holding final value
  spec_FuelT_t : FromWorkspace  VariableName=testSig_FuelT_t  Interpolate=off  OutputAfterFinalValue=Holding final value
  spec_GlwLmp_st : FromWorkspace  VariableName=testSig_GlwLmp_st  Interpolate=off  OutputAfterFinalValue=Holding final value
  spec_IAirHt_st : FromWorkspace  VariableName=testSig_IAirHt_st  Interpolate=off  OutputAfterFinalValue=Holding final value
  spec_Oil_tSwmp : FromWorkspace  VariableName=testSig_Oil_tSwmp  Interpolate=off  OutputAfterFinalValue=Holding final value
  spec_T15_st : FromWorkspace  VariableName=testSig_T15_st  Interpolate=off  OutputAfterFinalValue=Holding final value
  testSignals : Outport
  wires:
  BC/1 -> testSignals/1
  spec_T15_st/1 -> BC/1  "testSig_T15_st"
  spec_CoEng_st/1 -> BC/2  "testSig_CoEng_st"
  spec_Epm_nEng/1 -> BC/3  "testSig_Epm_nEng"
  spec_BattU_u/1 -> BC/4  "testSig_BattU_u"
  spec_CEngDsT_t/1 -> BC/5  "testSig_CEngDsT_t"
  spec_FuelT_t/1 -> BC/6  "testSig_FuelT_t"
  spec_Oil_tSwmp/1 -> BC/7  "testSig_Oil_tSwmp"
  spec_Air_tCACDs_mp/1 -> BC/8  "testSig_Air_tCACDs_mp"
  spec_Air_tAFS_mp/1 -> BC/9  "testSig_Air_tAFS_mp"
  spec_EnvT_t/1 -> BC/10  "testSig_EnvT_t"
  spec_Air_tIntkVUs/1 -> BC/11  "testSig_Air_tIntkVUs"
  spec_DSM_bAirHtCEngDsT/1 -> BC/12  "testSig_DSM_bAirHtCEngDsT"
  spec_DSM_bAirHtFuelT/1 -> BC/13  "testSig_DSM_bAirHtFuelT"
  spec_DSM_bAirHtOilT/1 -> BC/14  "testSig_DSM_bAirHtOilT"
  spec_DSM_bAirHtEnvT/1 -> BC/15  "testSig_DSM_bAirHtEnvT"
  spec_DSM_bAirHtCACDs/1 -> BC/16  "testSig_DSM_bAirHtCACDs"
  spec_DSM_bAirHtAFST/1 -> BC/17  "testSig_DSM_bAirHtAFST"
  spec_DSM_bAirHtIntkVUsT/1 -> BC/18  "testSig_DSM_bAirHtIntkVUsT"
  spec_AirHt_st/1 -> BC/19  "testSig_AirHt_st"
  spec_IAirHt_st/1 -> BC/20  "testSig_IAirHt_st"
  spec_GlwLmp_st/1 -> BC/21  "testSig_GlwLmp_st"

== system TST_AirHt_Ctl/simulationInput/testSignals_R004 ==
  BC : BusCreator  Inputs=21
  spec_AirHt_st : FromWorkspace  VariableName=testSig_AirHt_st  Interpolate=off  OutputAfterFinalValue=Holding final value
  spec_Air_tAFS_mp : FromWorkspace  VariableName=testSig_Air_tAFS_mp  Interpolate=off  OutputAfterFinalValue=Holding final value
  spec_Air_tCACDs_mp : FromWorkspace  VariableName=testSig_Air_tCACDs_mp  Interpolate=off  OutputAfterFinalValue=Holding final value
  spec_Air_tIntkVUs : FromWorkspace  VariableName=testSig_Air_tIntkVUs  Interpolate=off  OutputAfterFinalValue=Holding final value
  spec_BattU_u : FromWorkspace  VariableName=testSig_BattU_u  Interpolate=off  OutputAfterFinalValue=Holding final value
  spec_CEngDsT_t : FromWorkspace  VariableName=testSig_CEngDsT_t  Interpolate=off  OutputAfterFinalValue=Holding final value
  spec_CoEng_st : FromWorkspace  VariableName=testSig_CoEng_st  Interpolate=off  OutputAfterFinalValue=Holding final value
  spec_DSM_bAirHtAFST : FromWorkspace  VariableName=testSig_DSM_bAirHtAFST  Interpolate=off  OutputAfterFinalValue=Holding final value
  spec_DSM_bAirHtCACDs : FromWorkspace  VariableName=testSig_DSM_bAirHtCACDs  Interpolate=off  OutputAfterFinalValue=Holding final value
  spec_DSM_bAirHtCEngDsT : FromWorkspace  VariableName=testSig_DSM_bAirHtCEngDsT  Interpolate=off  OutputAfterFinalValue=Holding final value
  spec_DSM_bAirHtEnvT : FromWorkspace  VariableName=testSig_DSM_bAirHtEnvT  Interpolate=off  OutputAfterFinalValue=Holding final value
  spec_DSM_bAirHtFuelT : FromWorkspace  VariableName=testSig_DSM_bAirHtFuelT  Interpolate=off  OutputAfterFinalValue=Holding final value
  spec_DSM_bAirHtIntkVUsT : FromWorkspace  VariableName=testSig_DSM_bAirHtIntkVUsT  Interpolate=off  OutputAfterFinalValue=Holding final value
  spec_DSM_bAirHtOilT : FromWorkspace  VariableName=testSig_DSM_bAirHtOilT  Interpolate=off  OutputAfterFinalValue=Holding final value
  spec_EnvT_t : FromWorkspace  VariableName=testSig_EnvT_t  Interpolate=off  OutputAfterFinalValue=Holding final value
  spec_Epm_nEng : FromWorkspace  VariableName=testSig_Epm_nEng  Interpolate=off  OutputAfterFinalValue=Holding final value
  spec_FuelT_t : FromWorkspace  VariableName=testSig_FuelT_t  Interpolate=off  OutputAfterFinalValue=Holding final value
  spec_GlwLmp_st : FromWorkspace  VariableName=testSig_GlwLmp_st  Interpolate=off  OutputAfterFinalValue=Holding final value
  spec_IAirHt_st : FromWorkspace  VariableName=testSig_IAirHt_st  Interpolate=off  OutputAfterFinalValue=Holding final value
  spec_Oil_tSwmp : FromWorkspace  VariableName=testSig_Oil_tSwmp  Interpolate=off  OutputAfterFinalValue=Holding final value
  spec_T15_st : FromWorkspace  VariableName=testSig_T15_st  Interpolate=off  OutputAfterFinalValue=Holding final value
  testSignals : Outport
  wires:
  BC/1 -> testSignals/1
  spec_T15_st/1 -> BC/1  "testSig_T15_st"
  spec_CoEng_st/1 -> BC/2  "testSig_CoEng_st"
  spec_Epm_nEng/1 -> BC/3  "testSig_Epm_nEng"
  spec_BattU_u/1 -> BC/4  "testSig_BattU_u"
  spec_CEngDsT_t/1 -> BC/5  "testSig_CEngDsT_t"
  spec_FuelT_t/1 -> BC/6  "testSig_FuelT_t"
  spec_Oil_tSwmp/1 -> BC/7  "testSig_Oil_tSwmp"
  spec_Air_tCACDs_mp/1 -> BC/8  "testSig_Air_tCACDs_mp"
  spec_Air_tAFS_mp/1 -> BC/9  "testSig_Air_tAFS_mp"
  spec_EnvT_t/1 -> BC/10  "testSig_EnvT_t"
  spec_Air_tIntkVUs/1 -> BC/11  "testSig_Air_tIntkVUs"
  spec_DSM_bAirHtCEngDsT/1 -> BC/12  "testSig_DSM_bAirHtCEngDsT"
  spec_DSM_bAirHtFuelT/1 -> BC/13  "testSig_DSM_bAirHtFuelT"
  spec_DSM_bAirHtOilT/1 -> BC/14  "testSig_DSM_bAirHtOilT"
  spec_DSM_bAirHtEnvT/1 -> BC/15  "testSig_DSM_bAirHtEnvT"
  spec_DSM_bAirHtCACDs/1 -> BC/16  "testSig_DSM_bAirHtCACDs"
  spec_DSM_bAirHtAFST/1 -> BC/17  "testSig_DSM_bAirHtAFST"
  spec_DSM_bAirHtIntkVUsT/1 -> BC/18  "testSig_DSM_bAirHtIntkVUsT"
  spec_AirHt_st/1 -> BC/19  "testSig_AirHt_st"
  spec_IAirHt_st/1 -> BC/20  "testSig_IAirHt_st"
  spec_GlwLmp_st/1 -> BC/21  "testSig_GlwLmp_st"

== system TST_AirHt_Ctl/simulationInput/testSignals_R005 ==
  BC : BusCreator  Inputs=21
  spec_AirHt_st : FromWorkspace  VariableName=testSig_AirHt_st  Interpolate=off  OutputAfterFinalValue=Holding final value
  spec_Air_tAFS_mp : FromWorkspace  VariableName=testSig_Air_tAFS_mp  Interpolate=off  OutputAfterFinalValue=Holding final value
  spec_Air_tCACDs_mp : FromWorkspace  VariableName=testSig_Air_tCACDs_mp  Interpolate=off  OutputAfterFinalValue=Holding final value
  spec_Air_tIntkVUs : FromWorkspace  VariableName=testSig_Air_tIntkVUs  Interpolate=off  OutputAfterFinalValue=Holding final value
  spec_BattU_u : FromWorkspace  VariableName=testSig_BattU_u  Interpolate=off  OutputAfterFinalValue=Holding final value
  spec_CEngDsT_t : FromWorkspace  VariableName=testSig_CEngDsT_t  Interpolate=off  OutputAfterFinalValue=Holding final value
  spec_CoEng_st : FromWorkspace  VariableName=testSig_CoEng_st  Interpolate=off  OutputAfterFinalValue=Holding final value
  spec_DSM_bAirHtAFST : FromWorkspace  VariableName=testSig_DSM_bAirHtAFST  Interpolate=off  OutputAfterFinalValue=Holding final value
  spec_DSM_bAirHtCACDs : FromWorkspace  VariableName=testSig_DSM_bAirHtCACDs  Interpolate=off  OutputAfterFinalValue=Holding final value
  spec_DSM_bAirHtCEngDsT : FromWorkspace  VariableName=testSig_DSM_bAirHtCEngDsT  Interpolate=off  OutputAfterFinalValue=Holding final value
  spec_DSM_bAirHtEnvT : FromWorkspace  VariableName=testSig_DSM_bAirHtEnvT  Interpolate=off  OutputAfterFinalValue=Holding final value
  spec_DSM_bAirHtFuelT : FromWorkspace  VariableName=testSig_DSM_bAirHtFuelT  Interpolate=off  OutputAfterFinalValue=Holding final value
  spec_DSM_bAirHtIntkVUsT : FromWorkspace  VariableName=testSig_DSM_bAirHtIntkVUsT  Interpolate=off  OutputAfterFinalValue=Holding final value
  spec_DSM_bAirHtOilT : FromWorkspace  VariableName=testSig_DSM_bAirHtOilT  Interpolate=off  OutputAfterFinalValue=Holding final value
  spec_EnvT_t : FromWorkspace  VariableName=testSig_EnvT_t  Interpolate=off  OutputAfterFinalValue=Holding final value
  spec_Epm_nEng : FromWorkspace  VariableName=testSig_Epm_nEng  Interpolate=off  OutputAfterFinalValue=Holding final value
  spec_FuelT_t : FromWorkspace  VariableName=testSig_FuelT_t  Interpolate=off  OutputAfterFinalValue=Holding final value
  spec_GlwLmp_st : FromWorkspace  VariableName=testSig_GlwLmp_st  Interpolate=off  OutputAfterFinalValue=Holding final value
  spec_IAirHt_st : FromWorkspace  VariableName=testSig_IAirHt_st  Interpolate=off  OutputAfterFinalValue=Holding final value
  spec_Oil_tSwmp : FromWorkspace  VariableName=testSig_Oil_tSwmp  Interpolate=off  OutputAfterFinalValue=Holding final value
  spec_T15_st : FromWorkspace  VariableName=testSig_T15_st  Interpolate=off  OutputAfterFinalValue=Holding final value
  testSignals : Outport
  wires:
  BC/1 -> testSignals/1
  spec_T15_st/1 -> BC/1  "testSig_T15_st"
  spec_CoEng_st/1 -> BC/2  "testSig_CoEng_st"
  spec_Epm_nEng/1 -> BC/3  "testSig_Epm_nEng"
  spec_BattU_u/1 -> BC/4  "testSig_BattU_u"
  spec_CEngDsT_t/1 -> BC/5  "testSig_CEngDsT_t"
  spec_FuelT_t/1 -> BC/6  "testSig_FuelT_t"
  spec_Oil_tSwmp/1 -> BC/7  "testSig_Oil_tSwmp"
  spec_Air_tCACDs_mp/1 -> BC/8  "testSig_Air_tCACDs_mp"
  spec_Air_tAFS_mp/1 -> BC/9  "testSig_Air_tAFS_mp"
  spec_EnvT_t/1 -> BC/10  "testSig_EnvT_t"
  spec_Air_tIntkVUs/1 -> BC/11  "testSig_Air_tIntkVUs"
  spec_DSM_bAirHtCEngDsT/1 -> BC/12  "testSig_DSM_bAirHtCEngDsT"
  spec_DSM_bAirHtFuelT/1 -> BC/13  "testSig_DSM_bAirHtFuelT"
  spec_DSM_bAirHtOilT/1 -> BC/14  "testSig_DSM_bAirHtOilT"
  spec_DSM_bAirHtEnvT/1 -> BC/15  "testSig_DSM_bAirHtEnvT"
  spec_DSM_bAirHtCACDs/1 -> BC/16  "testSig_DSM_bAirHtCACDs"
  spec_DSM_bAirHtAFST/1 -> BC/17  "testSig_DSM_bAirHtAFST"
  spec_DSM_bAirHtIntkVUsT/1 -> BC/18  "testSig_DSM_bAirHtIntkVUsT"
  spec_AirHt_st/1 -> BC/19  "testSig_AirHt_st"
  spec_IAirHt_st/1 -> BC/20  "testSig_IAirHt_st"
  spec_GlwLmp_st/1 -> BC/21  "testSig_GlwLmp_st"
